simulink model "sfcndemo_atmos"  (Simulink 6.0)
settings: Solver=ode1  StartTime=0.0  StopTime=1200  RelTol=1e-3
settings Model: RequirementInfo=9  Creator=The MathWorks Inc.  LastModifiedBy=batserve  ExtModeAutoUpdateStatusClock=off  BufferReuse=off
settings OptimizationCC: BlockReduction=off  BooleanDataType=off  InlineParams=on  InlineInvariantSignals=off  OptimizeBlockIOStorage=off  BufferReuse=off  ExpressionFolding=off  LocalBlockOutputs=off
settings DebuggingCC: CheckExecutionContextPreStartOutputMsg=on  CheckExecutionContextRuntimeOutputMsg=on  SolverPrmCheckMsg=none
settings HardwareCC: TargetUnknown=on
settings RTWCC: MakeCommand="make_rtw S_FUNCTIONS_LIB=\"-lf2c\" FC=g77 USER_OBJS=\"atmos.o\""  RetainRTWFile=on

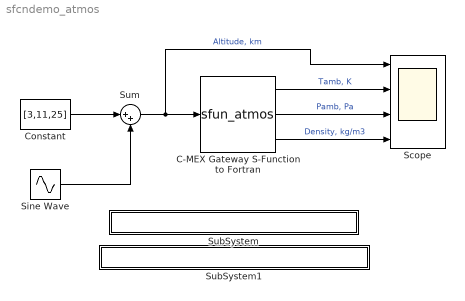
== system sfcndemo_atmos ==
  C-MEX Gateway S-Function to Fortran : S-Function  FunctionName=sfun_atmos  Parameters=288.15,101325.0,0.0103
  Constant : Constant  Value=[3,11,25]
  Scope : Scope  NumInputPorts=4
      settings: TimeRange=1200  YMin=0~200~0~0  YMax=30~300~150000~0.015
  Sine Wave : Sin  Amplitude=3  Frequency=0.01  SampleTime=0
  SubSystem : Subsystem  PropExecContextAcrossSSBoundary=on
      settings: OpenFcn=edit(fullfile(matlabroot,'simulink','src','sfun_atmos.c'))
      mask Display: disp('gateway: matlabroot\simulink\src\sfun_atmos.c');
  SubSystem1 : Subsystem  PropExecContextAcrossSSBoundary=on
      settings: OpenFcn=edit(fullfile(matlabroot,'simulink','src','sfun_atmos_sub.F'))
      mask Display: disp('Fortran: matlabroot\simulink\src\sfun_atmos_sub.f');
  Sum : Sum  Inputs=|++  SaturateOnIntegerOverflow=on  InputSameDT=on
  wires:
  Constant/1 -> Sum/1
  Sine Wave/1 -> Sum/2
  Sum/1 -> C-MEX Gateway S-Function to Fortran/1, Scope/1  "Altitude, km"
  C-MEX Gateway S-Function to Fortran/1 -> Scope/2  "Tamb, K"
  C-MEX Gateway S-Function to Fortran/2 -> Scope/3  "Pamb, Pa"
  C-MEX Gateway S-Function to Fortran/3 -> Scope/4  "Density, kg/m3"

== system sfcndemo_atmos/SubSystem ==

== system sfcndemo_atmos/SubSystem1 ==
